simulink model "MCC_P"  (R2025b)
settings: Solver=VariableStepAuto  StartTime=0.0  StopTime=4  RelTol=1e-3
undefined symbols (not defined in the file): cf, f, J, Ke, Kp, Kt, L, R, r
settings Model: Creator=$F3C000-T36KBJ93M5IO  LastModifiedBy=liset

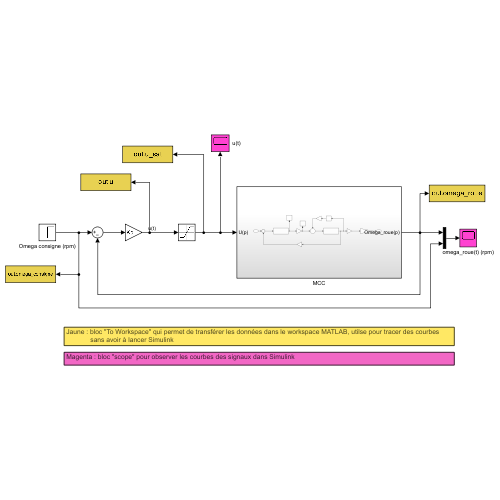
[thumbnail: Simulink's stored preview of the top-level diagram]
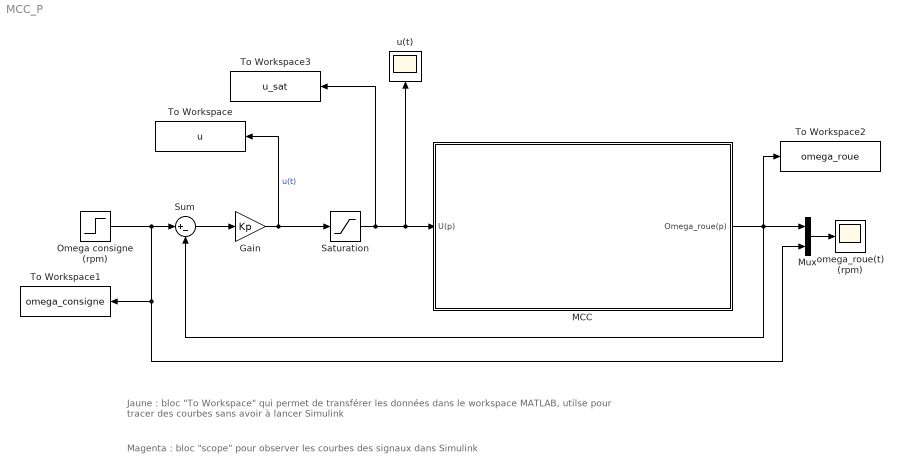
== system MCC_P ==
  note: Magenta : bloc "scope" pour observer les courbes des signaux dans Simulink
  note: Jaune : bloc "To Workspace" qui permet de transférer les données dans le workspace MATLAB, utilse pour tracer des courbes
      |              sans avoir à lancer Simulink
  Gain : Gain  Gain=Kp
  MCC : Subsystem
  Mux : Mux  Inputs=2
  Omega consigne (rpm) : Step  After=216  SampleTime=0
  Saturation : Saturate  UpperLimit=7.34  LowerLimit=-7.34
  Sum : Sum  Inputs=|+-
  To Workspace : ToWorkspace  VariableName=u  SampleTime=-1
  To Workspace1 : ToWorkspace  VariableName=omega_consigne  SampleTime=-1
  To Workspace2 : ToWorkspace  VariableName=omega_roue  SampleTime=-1
  To Workspace3 : ToWorkspace  VariableName=u_sat  SampleTime=-1
  omega_roue(t) (rpm) : Scope
      settings: ActiveDisplayYMinimum=30.932240726116788  ActiveDisplayYMaximum=349.87192239105997
  u(t) : Scope
      settings: ActiveDisplayYMinimum=-1  ActiveDisplayYMaximum=1  DataLoggingVariableName=ScopeData4
  wires:
  MCC/1(Omega_roue(p)) -> To Workspace2/1, Mux/1, Sum/2
  Omega consigne (rpm)/1 -> Sum/1, To Workspace1/1, Mux/2
  Sum/1 -> Gain/1
  Gain/1 -> Saturation/1, To Workspace/1  "u(t)"
  Mux/1 -> omega_roue(t) (rpm)/1
  Saturation/1 -> To Workspace3/1, u(t)/1, MCC/1(U(p))

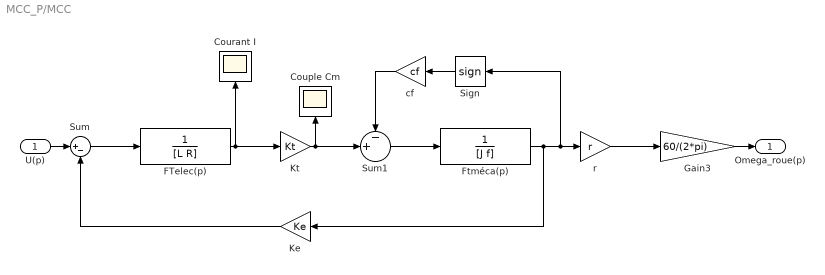
== system MCC_P/MCC ==
  U(p) : Inport
  Couple Cm : Scope
      settings: ActiveDisplayYMinimum=-1  ActiveDisplayYMaximum=1  DataLoggingVariableName=ScopeData2
  Courant I : Scope
      settings: ActiveDisplayYMinimum=-1  ActiveDisplayYMaximum=1
  FTelec(p) : TransferFcn  Denominator=[L R]
  Ftméca(p) : TransferFcn  Denominator=[J f]
  Gain3 : Gain  Gain=60/(2*pi)
  Ke : Gain  Gain=Ke
  Kt : Gain  Gain=Kt
  Sign : Signum
  Sum : Sum  Inputs=|+-
  Sum1 : Sum  Inputs=-+|
  cf : Gain  Gain=cf
  r : Gain  Gain=r
  Omega_roue(p) : Outport
  wires:
  Sum1/1 -> Ftméca(p)/1
  Sum/1 -> FTelec(p)/1
  Kt/1 -> Couple Cm/1, Sum1/2
  r/1 -> Gain3/1
  Ftméca(p)/1 -> r/1, Sign/1, Ke/1
  FTelec(p)/1 -> Kt/1, Courant I/1
  Ke/1 -> Sum/2
  Sign/1 -> cf/1
  cf/1 -> Sum1/1
  Gain3/1 -> Omega_roue(p)/1
  U(p)/1 -> Sum/1
